simulink library "WiFi_lib"  (Simulink 5.0)
values from neighbouring files (symbols this model uses):
  cck_codes_11 = [1 1 1 -1 1 1 -1 1 -1 1 -1 -1 ... (512 elements, 8x64)]    [cck_codes.mat]
  cck_codes_55 = [6.12303176911e-17 1 6.12303176911e-17 -1 6.12303176911e-17 1 -6.12303176911e-17 1 -1.83690953073e-16 1 -1.83690953073e-16 -1 ... (32 elements, 8x4)]    [cck_codes.mat]
  Center_frequency = (Channel_number-6) *5    [WiFi_init.m]
  Channel_size_change = 0    [WiFi_init.m]
  Correction_delay = evalin('base', 'Correction_delay')    [WiFi_init.m]
  Spreading_rate = evalin('base','Spreading_rate')    [WiFi_init.m]
undefined symbols (not defined in the file or in its folder): Buffering_delay, Chip_rate, PLCP_header_size, PLCP_preamble_size, PLCP_size, PLCP_size_symbols, PPDU_frame_period, PPDU_size_symbols, PSDU_size, PSDU_size_symbols
libraries: simulink x46, commdigbbndpm2 x17, dspsigattribs x14, simulink3 x14, WiFi_lib x14, dspmathops x8, dspmtrx3 x6, dspindex x4, dspsrcs3 x3, dspstat3 x2, commdigbbndfm2 x2, commchan2 x1
settings Model: Creator=stuartm  LastModifiedBy=stuartm

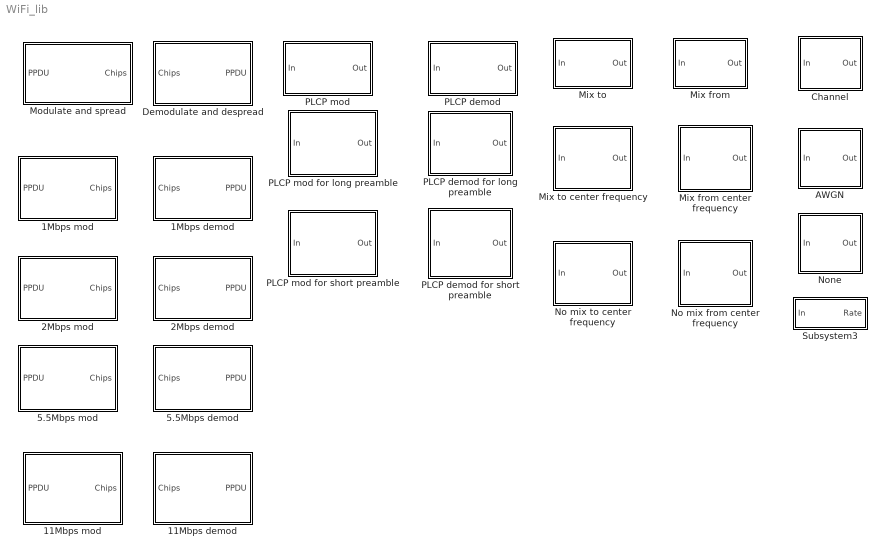
== system WiFi_lib ==
  11Mbps demod : Subsystem  mask{Short_preamble=off}
      mask prompts: Short_preamble "Short Preamble"
      mask init:
      | if Short_preamble
      |  set_param([gcb '/PLCP demod'],'BlockChoice','PLCP demod for short preamble')
      | else
      |   set_param([gcb '/PLCP demod'],'BlockChoice','PLCP demod for long preamble')
      | end
  11Mbps mod : Subsystem  mask{Short_preamble=off}
      mask prompts: Short_preamble "Short Preamble"
      mask init:
      | if Short_preamble
      |  set_param([gcb '/PLCP mod'],'BlockChoice','PLCP mod for short preamble')
      | else
      |   set_param([gcb '/PLCP mod'],'BlockChoice','PLCP mod for long preamble')
      | end
  1Mbps demod : Subsystem
  1Mbps mod : Subsystem
  2Mbps demod : Subsystem  mask{Short_preamble=off}
      mask prompts: Short_preamble "Short Preamble"
      mask init:
      | if Short_preamble
      |  set_param([gcb '/PLCP demod'],'BlockChoice','PLCP demod for short preamble')
      | else
      |   set_param([gcb '/PLCP demod'],'BlockChoice','PLCP demod for long preamble')
      | end
  2Mbps mod : Subsystem  mask{Short_preamble=off}
      mask prompts: Short_preamble "Short Preamble"
      mask init:
      | if Short_preamble
      |  set_param([gcb '/PLCP mod'],'BlockChoice','PLCP mod for short preamble')
      | else
      |   set_param([gcb '/PLCP mod'],'BlockChoice','PLCP mod for long preamble')
      | end
  5.5Mbps demod : Subsystem  mask{Short_preamble=off}
      mask prompts: Short_preamble "Short Preamble"
      mask init:
      | if Short_preamble
      |  set_param([gcb '/PLCP demod'],'BlockChoice','PLCP demod for short preamble')
      | else
      |   set_param([gcb '/PLCP demod'],'BlockChoice','PLCP demod for long preamble')
      | end
  5.5Mbps mod : Subsystem  mask{Short_preamble=off}
      mask prompts: Short_preamble "Short Preamble"
      mask init:
      | if Short_preamble
      |  set_param([gcb '/PLCP mod'],'BlockChoice','PLCP mod for short preamble')
      | else
      |   set_param([gcb '/PLCP mod'],'BlockChoice','PLCP mod for long preamble')
      | end
  AWGN : Subsystem
      mask Display: disp('Channel')
  Channel : Subsystem  BlockChoice=AWGN
      settings: TemplateBlock=self  MemberBlocks=AWGN,None
  Demodulate and despread : Subsystem  BlockChoice=11Mbps demod
      settings: TemplateBlock=self  MemberBlocks=11Mbps demod,1Mbps demod,2Mbps demod,5.5Mbps demod
  Mix from : Subsystem  BlockChoice=Mix from center frequency
      settings: TemplateBlock=self  MemberBlocks=Mix from center frequency,No mix from center frequency
  Mix from center frequency : Subsystem
  Mix to : Subsystem  BlockChoice=Mix to center frequency
      settings: TemplateBlock=self  MemberBlocks=Mix to center frequency,No mix to center frequency
  Mix to center frequency : Subsystem
  Modulate and spread : Subsystem  BlockChoice=11Mbps mod
      settings: TemplateBlock=self  MemberBlocks=11Mbps mod,1Mbps mod,2Mbps mod,5.5Mbps mod
  No mix from center frequency : Subsystem
  No mix to center frequency : Subsystem
  None : Subsystem
      mask Display: disp('Channel')
  PLCP demod : Subsystem  BlockChoice=PLCP demod for long preamble
      settings: TemplateBlock=self  MemberBlocks=PLCP demod for long preamble,PLCP demod for short preamble
  PLCP demod for long preamble : Subsystem
  PLCP demod for short preamble : Subsystem
  PLCP mod : Subsystem  BlockChoice=PLCP mod for long preamble
      settings: TemplateBlock=self  MemberBlocks=PLCP mod for long preamble,PLCP mod for short preamble
  PLCP mod for long preamble : Subsystem
  PLCP mod for short preamble : Subsystem
  Subsystem3 : Subsystem  mask(Display sample rate for framebased signals){Units=MHz}
      mask init:
      | switch Units
      | case 1
      |      Units_string='Hz';
      | case 2
      |      Units_string='KHz';
      | case 3
      |      Units_string='MHz';
      | end
      mask StyleString: popup(Hz|KHz|MHz)
      mask Display: disp(['Rate (' Units_string ')'])

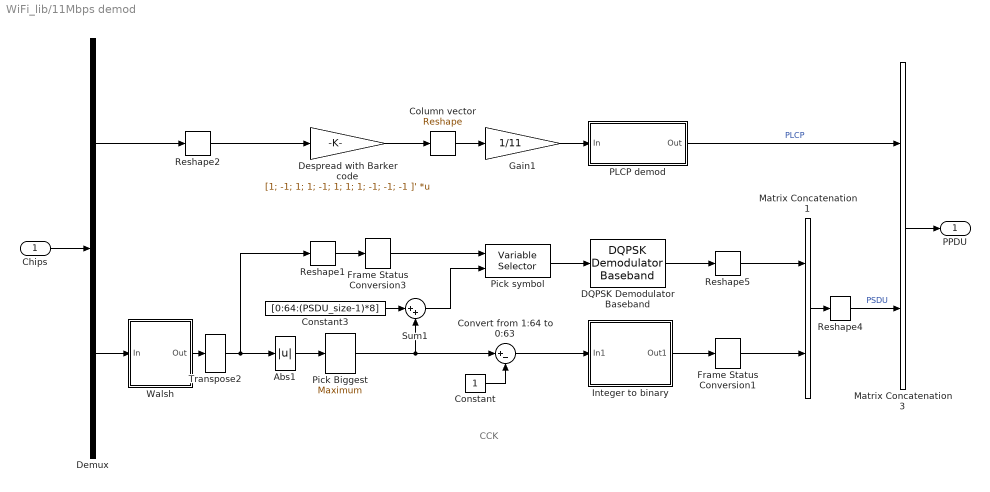
== system WiFi_lib/11Mbps demod ==
  note: CCK
  Chips : Inport
  Abs1 : Abs  SaturateOnIntegerOverflow=on
  Column vector : simulink/Math Operations/Reshape  OutputDimensionality=Column vector  OutputDimensions=[11,10]
  Constant : Constant
  Constant3 : Constant  Value=[0:64:(PSDU_size-1)*8]
  Convert from 1:64 to 0:63 : Sum  Inputs=|+-  SaturateOnIntegerOverflow=on  InputSameDT=on
  DQPSK Demodulator Baseband : commdigbbndpm2/DQPSK Demodulator Baseband  OutType=Bit  Dec=Binary  Ph=0  numSamp=1
  Demux : Demux  Outputs=[PLCP_size_symbols*Spreading_rate PSDU_size]
  Despread with Barker code : Gain  Gain=[1; -1; 1; 1; -1; 1; 1; 1; -1; -1; -1 ]'  Multiplication=Matrix(K*u)  SaturateOnIntegerOverflow=on
  Frame Status Conversion1 : dspsigattribs/Frame Status Conversion  growRefPort=off  outframe=Frame-based
  Frame Status Conversion3 : dspsigattribs/Frame Status Conversion  growRefPort=off  outframe=Frame-based
  Gain1 : Gain  Gain=1/11  SaturateOnIntegerOverflow=on
  Integer to binary : Subsystem
  Matrix Concatenation1 : simulink/Math Operations/Matrix Concatenation  numInports=2  catMethod=Vertical
  Matrix Concatenation3 : simulink/Math Operations/Matrix Concatenation  numInports=2  catMethod=Vertical
  PLCP demod : Subsystem  BlockChoice=PLCP demod for long preamble
      settings: AttributesFormatString=%<BlockChoice>  TemplateBlock=WiFi_lib/PLCP demod  MemberBlocks=PLCP demod for long preamble,PLCP demod for short preamble
  Pick Biggest : dspstat3/Maximum  fcn=Index  reset=None
  Pick symbol : dspindex/Variable Selector  rowsOrCols=Rows  IdxMode=Variable  Elements=[1 3]  ZerOneIdxMode=One-based  errmode=Clip Index
  Reshape1 : simulink/Math Operations/Reshape  OutputDimensionality=1-D array  OutputDimensions=[Spreading_rate,PLCP_size_symbols]
  Reshape2 : simulink/Math Operations/Reshape  OutputDimensionality=Customize  OutputDimensions=[Spreading_rate,PLCP_size_symbols]
  Reshape4 : simulink/Math Operations/Reshape  OutputDimensionality=Column vector  OutputDimensions=[Spreading_rate,PLCP_size_symbols]
  Reshape5 : simulink/Math Operations/Reshape  OutputDimensionality=Customize  OutputDimensions=[2,PSDU_size/8]
  Sum1 : Sum  Inputs=|++  SaturateOnIntegerOverflow=on  InputSameDT=on
  Transpose2 : dspmtrx3/Transpose  Hermitian=off
  Walsh : Subsystem
  PPDU : Outport
  wires:
  Gain1/1 -> PLCP demod/1(In)
  Despread with Barker code/1 -> Column vector/1
  Column vector/1 -> Gain1/1
  Demux/1 -> Reshape2/1
  Demux/2 -> Walsh/1(In)
  Chips/1 -> Demux/1
  PLCP demod/1(Out) -> Matrix Concatenation3/1  "PLCP"
  Reshape4/1 -> Matrix Concatenation3/2  "PSDU"
  Matrix Concatenation3/1 -> PPDU/1
  Walsh/1(Out) -> Transpose2/1
  Transpose2/1 -> Abs1/1, Reshape1/1
  Abs1/1 -> Pick Biggest/1
  Pick Biggest/1 -> Convert from 1:64 to 0:63/1, Sum1/2
  Constant/1 -> Convert from 1:64 to 0:63/2
  Convert from 1:64 to 0:63/1 -> Integer to binary/1(In1)
  Integer to binary/1(Out1) -> Frame Status Conversion1/1
  Pick symbol/1 -> DQPSK Demodulator Baseband/1
  Reshape5/1 -> Matrix Concatenation1/1
  Reshape1/1 -> Frame Status Conversion3/1
  Sum1/1 -> Pick symbol/2
  Constant3/1 -> Sum1/1
  Frame Status Conversion1/1 -> Matrix Concatenation1/2
  Frame Status Conversion3/1 -> Pick symbol/1
  Matrix Concatenation1/1 -> Reshape4/1
  DQPSK Demodulator Baseband/1 -> Reshape5/1
  Reshape2/1 -> Despread with Barker code/1

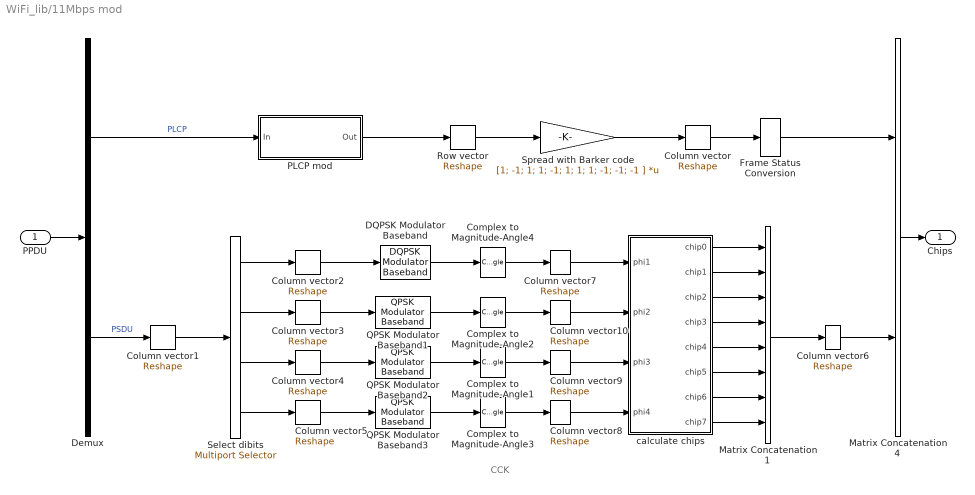
== system WiFi_lib/11Mbps mod ==
  note: CCK
  PPDU : Inport
  Column vector : simulink/Math Operations/Reshape  OutputDimensionality=Column vector  OutputDimensions=[1,1]
  Column vector1 : simulink/Math Operations/Reshape  OutputDimensionality=Customize  OutputDimensions=[8,PSDU_size/8]
  Column vector{7..10} (4 alike) : simulink/Math Operations/Reshape  OutputDimensionality=Row vector  OutputDimensions=[8,PSDU_size/8]
  Column vector{2..6} (5 alike) : simulink/Math Operations/Reshape  OutputDimensionality=Column vector  OutputDimensions=[8,PSDU_size/8]
  Complex to Magnitude-Angle{1..4} (4 alike) : ComplexToMagnitudeAngle  Output=Angle
  DQPSK Modulator Baseband : commdigbbndpm2/DQPSK Modulator Baseband  InType=Bit  Enc=Binary  Ph=0  numSamp=1
  Demux : Demux  Outputs=[PLCP_size PSDU_size]
  Frame Status Conversion : dspsigattribs/Frame Status Conversion  growRefPort=off  outframe=Frame-based
  Matrix Concatenation1 : simulink/Math Operations/Matrix Concatenation  numInports=8  catMethod=Vertical
  Matrix Concatenation4 : simulink/Math Operations/Matrix Concatenation  numInports=2  catMethod=Vertical
  PLCP mod : Subsystem  BlockChoice=PLCP mod for long preamble
      settings: AttributesFormatString=%<BlockChoice>  TemplateBlock=WiFi_lib/PLCP mod  MemberBlocks=PLCP mod for long preamble,PLCP mod for short preamble
  QPSK Modulator Baseband1 : commdigbbndpm2/QPSK Modulator Baseband  InType=Bit  Enc=Binary  Ph=0  numSamp=1
  QPSK Modulator Baseband2 : commdigbbndpm2/QPSK Modulator Baseband  InType=Bit  Enc=Binary  Ph=0  numSamp=1
  QPSK Modulator Baseband3 : commdigbbndpm2/QPSK Modulator Baseband  InType=Bit  Enc=Binary  Ph=0  numSamp=1
  Row vector : simulink/Math Operations/Reshape  OutputDimensionality=Row vector  OutputDimensions=[1,1]
  Select dibits : dspindex/Multiport Selector  rowsOrCols=Rows  idxCellArray={ [1 2], [3 4], [5 6], [ 7 8] }  idxErrMode=Generate Error
  Spread with Barker code : Gain  Gain=[1; -1; 1; 1; -1; 1; 1; 1; -1; -1; -1 ]  Multiplication=Matrix(K*u)  SaturateOnIntegerOverflow=on
  calculate chips : Subsystem
  Chips : Outport
  wires:
  Column vector6/1 -> Matrix Concatenation4/2
  PLCP mod/1(Out) -> Row vector/1
  Spread with Barker code/1 -> Column vector/1
  Column vector/1 -> Frame Status Conversion/1
  Frame Status Conversion/1 -> Matrix Concatenation4/1
  Matrix Concatenation4/1 -> Chips/1
  PPDU/1 -> Demux/1
  Demux/1 -> PLCP mod/1(In)  "PLCP"
  Demux/2 -> Column vector1/1  "PSDU"
  Column vector1/1 -> Select dibits/1
  Select dibits/1 -> Column vector2/1
  Select dibits/2 -> Column vector3/1
  Select dibits/3 -> Column vector4/1
  Select dibits/4 -> Column vector5/1
  Column vector2/1 -> DQPSK Modulator Baseband/1
  Column vector3/1 -> QPSK Modulator Baseband1/1
  Column vector4/1 -> QPSK Modulator Baseband2/1
  Column vector5/1 -> QPSK Modulator Baseband3/1
  DQPSK Modulator Baseband/1 -> Complex to Magnitude-Angle4/1
  QPSK Modulator Baseband1/1 -> Complex to Magnitude-Angle2/1
  QPSK Modulator Baseband2/1 -> Complex to Magnitude-Angle1/1
  QPSK Modulator Baseband3/1 -> Complex to Magnitude-Angle3/1
  Complex to Magnitude-Angle4/1 -> Column vector7/1
  Complex to Magnitude-Angle2/1 -> Column vector10/1
  Complex to Magnitude-Angle1/1 -> Column vector9/1
  Complex to Magnitude-Angle3/1 -> Column vector8/1
  calculate chips/2(chip1) -> Matrix Concatenation1/2
  calculate chips/3(chip2) -> Matrix Concatenation1/3
  calculate chips/4(chip3) -> Matrix Concatenation1/4
  calculate chips/5(chip4) -> Matrix Concatenation1/5
  calculate chips/6(chip5) -> Matrix Concatenation1/6
  calculate chips/7(chip6) -> Matrix Concatenation1/7
  calculate chips/8(chip7) -> Matrix Concatenation1/8
  Matrix Concatenation1/1 -> Column vector6/1
  Column vector8/1 -> calculate chips/4(phi4)
  Column vector9/1 -> calculate chips/3(phi3)
  Column vector10/1 -> calculate chips/2(phi2)
  Column vector7/1 -> calculate chips/1(phi1)
  calculate chips/1(chip0) -> Matrix Concatenation1/1
  Row vector/1 -> Spread with Barker code/1

== system WiFi_lib/1Mbps demod ==
  Chips : Inport
  Column vector : simulink/Math Operations/Reshape  OutputDimensionality=Column vector  OutputDimensions=[11,10]
  DBPSK Demodulator Baseband : commdigbbndpm2/DBPSK Demodulator Baseband  Ph=0  numSamp=1
  Despread with Barker code : Gain  Gain=[1; -1; 1; 1; -1; 1; 1; 1; -1; -1; -1 ]'  Multiplication=Matrix(K*u)  SaturateOnIntegerOverflow=on
  Gain1 : Gain  Gain=1/11  SaturateOnIntegerOverflow=on
  Reshape2 : simulink/Math Operations/Reshape  OutputDimensionality=Customize  OutputDimensions=[Spreading_rate,PPDU_size_symbols]
  PPDU : Outport
  wires:
  DBPSK Demodulator Baseband/1 -> PPDU/1
  Chips/1 -> Reshape2/1
  Column vector/1 -> Gain1/1
  Despread with Barker code/1 -> Column vector/1
  Gain1/1 -> DBPSK Demodulator Baseband/1
  Reshape2/1 -> Despread with Barker code/1

== system WiFi_lib/1Mbps mod ==
  PPDU : Inport
  Column vector : simulink/Math Operations/Reshape  OutputDimensionality=Column vector  OutputDimensions=[1,1]
  DBPSK Modulator Baseband1 : commdigbbndpm2/DBPSK Modulator Baseband  Ph=0  numSamp=1
  Frame Status Conversion : dspsigattribs/Frame Status Conversion  growRefPort=off  outframe=Frame-based
  Row vector : simulink/Math Operations/Reshape  OutputDimensionality=Row vector  OutputDimensions=[1,1]
  Spread with Barker code : Gain  Gain=[1; -1; 1; 1; -1; 1; 1; 1; -1; -1; -1 ]  Multiplication=Matrix(K*u)  SaturateOnIntegerOverflow=on
  Chips : Outport
  wires:
  DBPSK Modulator Baseband1/1 -> Row vector/1
  Spread with Barker code/1 -> Column vector/1
  Column vector/1 -> Frame Status Conversion/1  "PPDU"
  PPDU/1 -> DBPSK Modulator Baseband1/1
  Frame Status Conversion/1 -> Chips/1  "PPDU"
  Row vector/1 -> Spread with Barker code/1

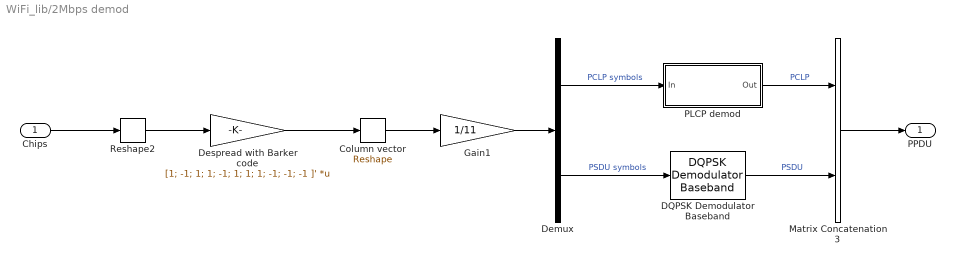
== system WiFi_lib/2Mbps demod ==
  Chips : Inport
  Column vector : simulink/Math Operations/Reshape  OutputDimensionality=Column vector  OutputDimensions=[11,10]
  DQPSK Demodulator Baseband : commdigbbndpm2/DQPSK Demodulator Baseband  OutType=Bit  Dec=Gray  Ph=0  numSamp=1
  Demux : Demux  Outputs=[PLCP_size_symbols PSDU_size_symbols]
  Despread with Barker code : Gain  Gain=[1; -1; 1; 1; -1; 1; 1; 1; -1; -1; -1 ]'  Multiplication=Matrix(K*u)  SaturateOnIntegerOverflow=on
  Gain1 : Gain  Gain=1/11  SaturateOnIntegerOverflow=on
  Matrix Concatenation3 : simulink/Math Operations/Matrix Concatenation  numInports=2  catMethod=Vertical
  PLCP demod : Subsystem  BlockChoice=PLCP demod for long preamble
      settings: AttributesFormatString=%<BlockChoice>  TemplateBlock=WiFi_lib/PLCP demod  MemberBlocks=PLCP demod for long preamble,PLCP demod for short preamble
  Reshape2 : simulink/Math Operations/Reshape  OutputDimensionality=Customize  OutputDimensions=[Spreading_rate,PPDU_size_symbols]
  PPDU : Outport
  wires:
  PLCP demod/1(Out) -> Matrix Concatenation3/1  "PCLP"
  Demux/1 -> PLCP demod/1(In)  "PCLP symbols"
  Demux/2 -> DQPSK Demodulator Baseband/1  "PSDU symbols"
  Gain1/1 -> Demux/1
  Despread with Barker code/1 -> Column vector/1
  Column vector/1 -> Gain1/1
  Chips/1 -> Reshape2/1
  Matrix Concatenation3/1 -> PPDU/1
  DQPSK Demodulator Baseband/1 -> Matrix Concatenation3/2  "PSDU"
  Reshape2/1 -> Despread with Barker code/1

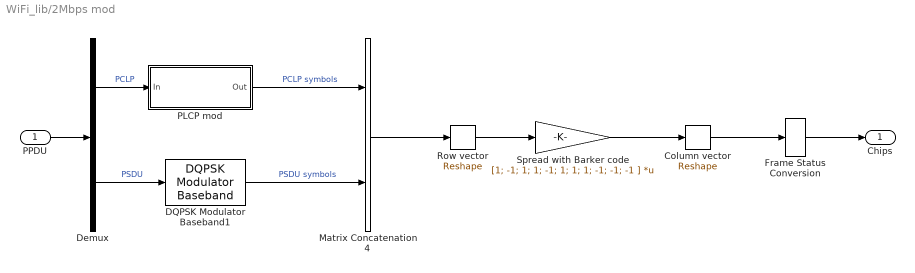
== system WiFi_lib/2Mbps mod ==
  PPDU : Inport
  Column vector : simulink/Math Operations/Reshape  OutputDimensionality=Column vector  OutputDimensions=[1,1]
  DQPSK Modulator Baseband1 : commdigbbndpm2/DQPSK Modulator Baseband  InType=Bit  Enc=Gray  Ph=0  numSamp=1
  Demux : Demux  Outputs=[PLCP_size PSDU_size]
  Frame Status Conversion : dspsigattribs/Frame Status Conversion  growRefPort=off  outframe=Frame-based
  Matrix Concatenation4 : simulink/Math Operations/Matrix Concatenation  numInports=2  catMethod=Vertical
  PLCP mod : Subsystem  BlockChoice=PLCP mod for long preamble
      settings: AttributesFormatString=%<BlockChoice>  TemplateBlock=WiFi_lib/PLCP mod  MemberBlocks=PLCP mod for long preamble,PLCP mod for short preamble
  Row vector : simulink/Math Operations/Reshape  OutputDimensionality=Row vector  OutputDimensions=[1,1]
  Spread with Barker code : Gain  Gain=[1; -1; 1; 1; -1; 1; 1; 1; -1; -1; -1 ]  Multiplication=Matrix(K*u)  SaturateOnIntegerOverflow=on
  Chips : Outport
  wires:
  Spread with Barker code/1 -> Column vector/1
  Column vector/1 -> Frame Status Conversion/1
  Frame Status Conversion/1 -> Chips/1
  PLCP mod/1(Out) -> Matrix Concatenation4/1  "PCLP symbols"
  Matrix Concatenation4/1 -> Row vector/1
  DQPSK Modulator Baseband1/1 -> Matrix Concatenation4/2  "PSDU symbols"
  Demux/1 -> PLCP mod/1(In)  "PCLP"
  PPDU/1 -> Demux/1
  Demux/2 -> DQPSK Modulator Baseband1/1  "PSDU"
  Row vector/1 -> Spread with Barker code/1

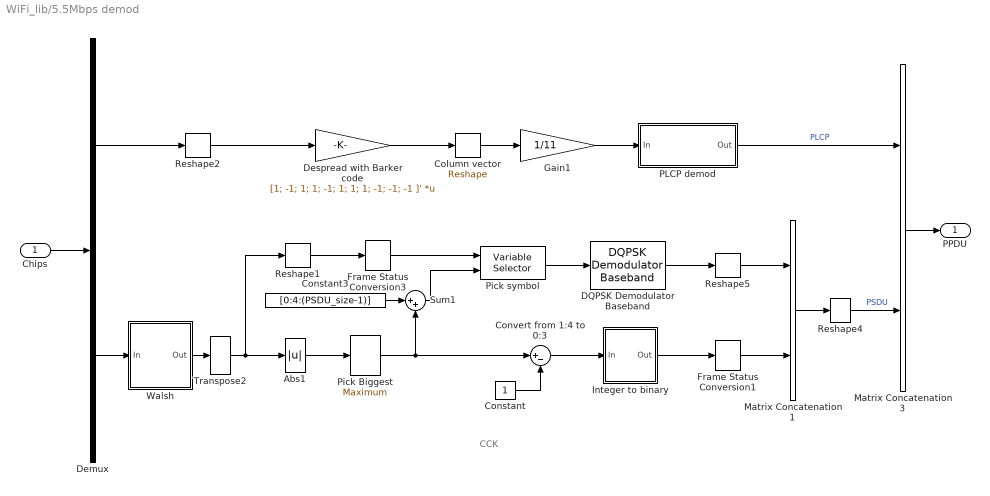
== system WiFi_lib/5.5Mbps demod ==
  note: CCK
  Chips : Inport
  Abs1 : Abs  SaturateOnIntegerOverflow=on
  Column vector : simulink/Math Operations/Reshape  OutputDimensionality=Column vector  OutputDimensions=[11,10]
  Constant : Constant
  Constant3 : Constant  Value=[0:4:(PSDU_size-1)]
  Convert from 1:4 to 0:3 : Sum  Inputs=|+-  SaturateOnIntegerOverflow=on  InputSameDT=on
  DQPSK Demodulator Baseband : commdigbbndpm2/DQPSK Demodulator Baseband  OutType=Bit  Dec=Binary  Ph=0  numSamp=1
  Demux : Demux  Outputs=[PLCP_size_symbols*Spreading_rate PSDU_size*2]
  Despread with Barker code : Gain  Gain=[1; -1; 1; 1; -1; 1; 1; 1; -1; -1; -1 ]'  Multiplication=Matrix(K*u)  SaturateOnIntegerOverflow=on
  Frame Status Conversion1 : dspsigattribs/Frame Status Conversion  growRefPort=off  outframe=Frame-based
  Frame Status Conversion3 : dspsigattribs/Frame Status Conversion  growRefPort=off  outframe=Frame-based
  Gain1 : Gain  Gain=1/11  SaturateOnIntegerOverflow=on
  Integer to binary : Subsystem
  Matrix Concatenation1 : simulink/Math Operations/Matrix Concatenation  numInports=2  catMethod=Vertical
  Matrix Concatenation3 : simulink/Math Operations/Matrix Concatenation  numInports=2  catMethod=Vertical
  PLCP demod : Subsystem  BlockChoice=PLCP demod for long preamble
      settings: AttributesFormatString=%<BlockChoice>  TemplateBlock=WiFi_lib/PLCP demod  MemberBlocks=PLCP demod for long preamble,PLCP demod for short preamble
  Pick Biggest : dspstat3/Maximum  fcn=Index  reset=None
  Pick symbol : dspindex/Variable Selector  rowsOrCols=Rows  IdxMode=Variable  Elements=[1 3]  ZerOneIdxMode=One-based  errmode=Clip Index
  Reshape1 : simulink/Math Operations/Reshape  OutputDimensionality=1-D array  OutputDimensions=[Spreading_rate,PLCP_size_symbols]
  Reshape2 : simulink/Math Operations/Reshape  OutputDimensionality=Customize  OutputDimensions=[Spreading_rate,PLCP_size_symbols]
  Reshape4 : simulink/Math Operations/Reshape  OutputDimensionality=Column vector  OutputDimensions=[Spreading_rate,PLCP_size_symbols]
  Reshape5 : simulink/Math Operations/Reshape  OutputDimensionality=Customize  OutputDimensions=[2,PSDU_size/4]
  Sum1 : Sum  Inputs=|++  SaturateOnIntegerOverflow=on  InputSameDT=on
  Transpose2 : dspmtrx3/Transpose  Hermitian=off
  Walsh : Subsystem
  PPDU : Outport
  wires:
  DQPSK Demodulator Baseband/1 -> Reshape5/1
  Matrix Concatenation1/1 -> Reshape4/1
  Frame Status Conversion3/1 -> Pick symbol/1
  Frame Status Conversion1/1 -> Matrix Concatenation1/2
  Constant3/1 -> Sum1/1
  Sum1/1 -> Pick symbol/2
  Reshape1/1 -> Frame Status Conversion3/1
  Reshape5/1 -> Matrix Concatenation1/1
  Pick symbol/1 -> DQPSK Demodulator Baseband/1
  Integer to binary/1(Out) -> Frame Status Conversion1/1
  Convert from 1:4 to 0:3/1 -> Integer to binary/1(In)
  Constant/1 -> Convert from 1:4 to 0:3/2
  Pick Biggest/1 -> Sum1/2, Convert from 1:4 to 0:3/1
  Abs1/1 -> Pick Biggest/1
  Transpose2/1 -> Abs1/1, Reshape1/1
  Walsh/1(Out) -> Transpose2/1
  Matrix Concatenation3/1 -> PPDU/1
  Reshape4/1 -> Matrix Concatenation3/2  "PSDU"
  PLCP demod/1(Out) -> Matrix Concatenation3/1  "PLCP"
  Chips/1 -> Demux/1
  Demux/2 -> Walsh/1(In)
  Demux/1 -> Reshape2/1
  Column vector/1 -> Gain1/1
  Despread with Barker code/1 -> Column vector/1
  Gain1/1 -> PLCP demod/1(In)
  Reshape2/1 -> Despread with Barker code/1

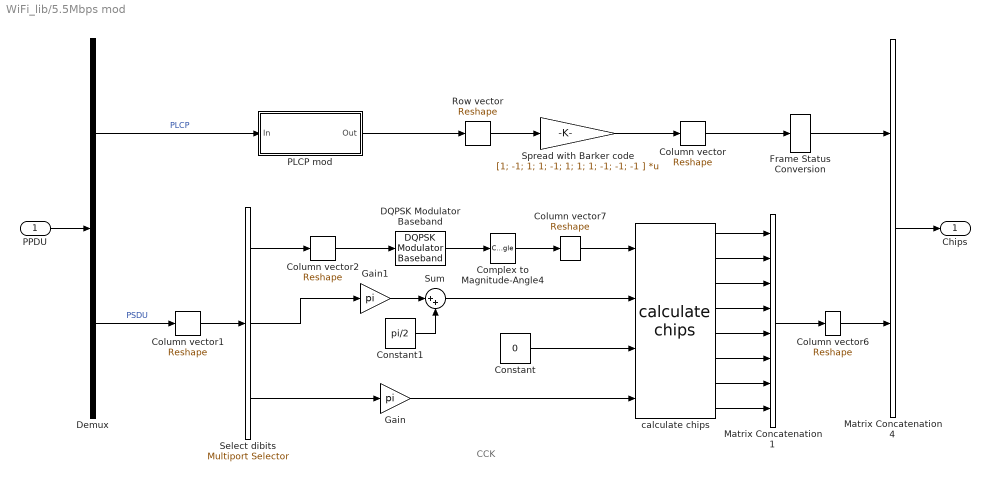
== system WiFi_lib/5.5Mbps mod ==
  note: CCK
  PPDU : Inport
  Column vector : simulink/Math Operations/Reshape  OutputDimensionality=Column vector  OutputDimensions=[1,1]
  Column vector1 : simulink/Math Operations/Reshape  OutputDimensionality=Customize  OutputDimensions=[4,PSDU_size/4]
  Column vector2 : simulink/Math Operations/Reshape  OutputDimensionality=Column vector  OutputDimensions=[8,PSDU_size/8]
  Column vector6 : simulink/Math Operations/Reshape  OutputDimensionality=Column vector  OutputDimensions=[8,PSDU_size/8]
  Column vector7 : simulink/Math Operations/Reshape  OutputDimensionality=Row vector  OutputDimensions=[8,PSDU_size/8]
  Complex to Magnitude-Angle4 : ComplexToMagnitudeAngle  Output=Angle
  Constant : Constant  Value=0
  Constant1 : Constant  Value=pi/2
  DQPSK Modulator Baseband : commdigbbndpm2/DQPSK Modulator Baseband  InType=Bit  Enc=Binary  Ph=0  numSamp=1
  Demux : Demux  Outputs=[PLCP_size PSDU_size]
  Frame Status Conversion : dspsigattribs/Frame Status Conversion  growRefPort=off  outframe=Frame-based
  Gain : Gain  Gain=pi  SaturateOnIntegerOverflow=on
  Gain1 : Gain  Gain=pi  SaturateOnIntegerOverflow=on
  Matrix Concatenation1 : simulink/Math Operations/Matrix Concatenation  numInports=8  catMethod=Vertical
  Matrix Concatenation4 : simulink/Math Operations/Matrix Concatenation  numInports=2  catMethod=Vertical
  PLCP mod : Subsystem  BlockChoice=PLCP mod for long preamble
      settings: AttributesFormatString=%<BlockChoice>  TemplateBlock=WiFi_lib/PLCP mod  MemberBlocks=PLCP mod for long preamble,PLCP mod for short preamble
  Row vector : simulink/Math Operations/Reshape  OutputDimensionality=Row vector  OutputDimensions=[1,1]
  Select dibits : dspindex/Multiport Selector  rowsOrCols=Rows  idxCellArray={ [1 2], 3,4}  idxErrMode=Generate Error
  Spread with Barker code : Gain  Gain=[1; -1; 1; 1; -1; 1; 1; 1; -1; -1; -1 ]  Multiplication=Matrix(K*u)  SaturateOnIntegerOverflow=on
  Sum : Sum  Inputs=|++  SaturateOnIntegerOverflow=on  InputSameDT=on
  calculate chips : WiFi_lib/11Mbps mod/calculate chips  SimViewingDevice=off  DataTypeOverride=UseLocalSettings  MinMaxOverflowLogging=UseLocalSettings
      settings: Permissions=ReadWrite  RTWFcnNameOpts=Auto  RTWFileNameOpts=Auto
  Chips : Outport
  wires:
  Column vector6/1 -> Matrix Concatenation4/2
  PLCP mod/1(Out) -> Row vector/1
  Demux/1 -> PLCP mod/1(In)  "PLCP"
  Spread with Barker code/1 -> Column vector/1
  Column vector/1 -> Frame Status Conversion/1
  Frame Status Conversion/1 -> Matrix Concatenation4/1
  Matrix Concatenation4/1 -> Chips/1
  Demux/2 -> Column vector1/1  "PSDU"
  PPDU/1 -> Demux/1
  Column vector1/1 -> Select dibits/1
  Select dibits/1 -> Column vector2/1
  Column vector2/1 -> DQPSK Modulator Baseband/1
  DQPSK Modulator Baseband/1 -> Complex to Magnitude-Angle4/1
  Complex to Magnitude-Angle4/1 -> Column vector7/1
  calculate chips/2 -> Matrix Concatenation1/2
  calculate chips/3 -> Matrix Concatenation1/3
  calculate chips/4 -> Matrix Concatenation1/4
  calculate chips/5 -> Matrix Concatenation1/5
  calculate chips/6 -> Matrix Concatenation1/6
  calculate chips/7 -> Matrix Concatenation1/7
  calculate chips/8 -> Matrix Concatenation1/8
  Matrix Concatenation1/1 -> Column vector6/1
  Column vector7/1 -> calculate chips/1
  calculate chips/1 -> Matrix Concatenation1/1
  Gain/1 -> calculate chips/4
  Constant/1 -> calculate chips/3
  Gain1/1 -> Sum/1
  Constant1/1 -> Sum/2
  Sum/1 -> calculate chips/2
  Select dibits/2 -> Gain1/1
  Select dibits/3 -> Gain/1
  Row vector/1 -> Spread with Barker code/1

== system WiFi_lib/AWGN ==
  In : Inport
  AWGN Channel : commchan2/AWGN Channel  seed=1237  noiseMode="Signal to noise ratio  (Es/No)"  EsNodB=EsNo  SNRdB=10  Ps=1  Tsym=1/Chip_rate  variance=1
  Out : Outport
  wires:
  AWGN Channel/1 -> Out/1
  In/1 -> AWGN Channel/1

== system WiFi_lib/Channel ==
  In : Inport
  AWGN : WiFi_lib/AWGN
  Out : Outport
  wires:
  In/1 -> AWGN/1
  AWGN/1 -> Out/1

== system WiFi_lib/Demodulate and despread ==
  Chips : Inport
  11Mbps demod : WiFi_lib/11Mbps demod  Short_preamble=off
  PPDU : Outport
  wires:
  Chips/1 -> 11Mbps demod/1
  11Mbps demod/1 -> PPDU/1

== system WiFi_lib/Mix from ==
  In : Inport
  Mix from center frequency : WiFi_lib/Mix from center frequency
      settings: RTWFcnNameOpts=Auto  RTWFileNameOpts=Auto
  Out : Outport
  wires:
  In/1 -> Mix from center frequency/1
  Mix from center frequency/1 -> Out/1

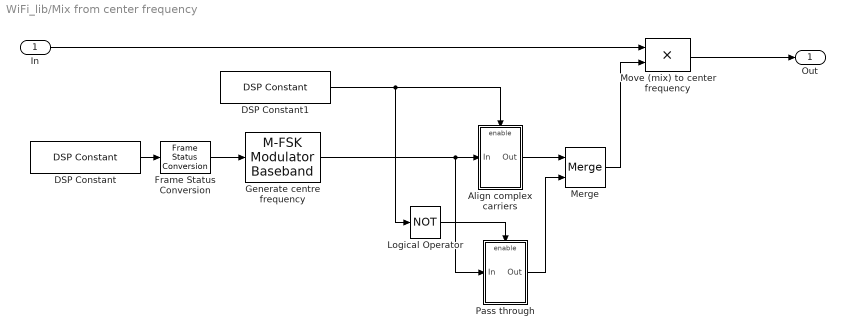
== system WiFi_lib/Mix from center frequency ==
  In : Inport
  Align complex carriers : Subsystem  TreatAsAtomicUnit=on
  DSP Constant : dspsrcs3/DSP Constant  Value=-Center_frequency+39  InterpretAs1D=off  SampleMode=Discrete  Ts=PPDU_frame_period/8  FramebasedOutput=off
  DSP Constant1 : dspsrcs3/DSP Constant  Value=Channel_size_change  InterpretAs1D=off  SampleMode=Discrete  Ts=PPDU_frame_period/8  FramebasedOutput=off
  Frame Status Conversion : dspsigattribs/Frame Status Conversion  growRefPort=off  outframe=Frame-based
  "Generate centre frequency " : commdigbbndfm2/M-FSK Modulator Baseband  M=79  InType=Integer  Enc=Binary  freqSep=1e6  phaseType=Continuous  numSamp=PPDU_size_chips
  Logical Operator : Logic  Operator=NOT
  Merge : Merge
  Move (mix) to center frequency : Product  SaturateOnIntegerOverflow=on  InputSameDT=on
  Pass through : Subsystem  TreatAsAtomicUnit=on
  Out : Outport
  wires:
  Frame Status Conversion/1 -> "Generate centre frequency "/1
  DSP Constant/1 -> Frame Status Conversion/1
  In/1 -> Move (mix) to center frequency/1
  Move (mix) to center frequency/1 -> Out/1
  "Generate centre frequency "/1 -> Align complex carriers/1(In), Pass through/1(In)
  DSP Constant1/1 -> Align complex carriers/Enable, Logical Operator/1
  Logical Operator/1 -> Pass through/Enable
  Align complex carriers/1(Out) -> Merge/1
  Pass through/1(Out) -> Merge/2
  Merge/1 -> Move (mix) to center frequency/2

== system WiFi_lib/Mix to ==
  In : Inport
  Mix to center frequency : WiFi_lib/Mix to center frequency
      settings: RTWFcnNameOpts=Auto  RTWFileNameOpts=Auto
  Out : Outport
  wires:
  In/1 -> Mix to center frequency/1
  Mix to center frequency/1 -> Out/1

== system WiFi_lib/Mix to center frequency ==
  In : Inport
  DSP Constant : dspsrcs3/DSP Constant  Value=Center_frequency+39  InterpretAs1D=off  SampleMode=Discrete  Ts=PPDU_frame_period/8  FramebasedOutput=off
  Frame Status Conversion : dspsigattribs/Frame Status Conversion  growRefPort=off  outframe=Frame-based
  "Generate centre frequency " : commdigbbndfm2/M-FSK Modulator Baseband  M=79  InType=Integer  Enc=Binary  freqSep=1e6  phaseType=Continuous  numSamp=PPDU_size_chips
  Move center frequency : Product  SaturateOnIntegerOverflow=on  InputSameDT=on
  Out : Outport
  wires:
  Move center frequency/1 -> Out/1
  In/1 -> Move center frequency/1
  DSP Constant/1 -> Frame Status Conversion/1
  "Generate centre frequency "/1 -> Move center frequency/2
  Frame Status Conversion/1 -> "Generate centre frequency "/1

== system WiFi_lib/Modulate and spread ==
  PPDU : Inport
  11Mbps mod : WiFi_lib/11Mbps mod  Short_preamble=off
  Chips : Outport
  wires:
  PPDU/1 -> 11Mbps mod/1
  11Mbps mod/1 -> Chips/1

== system WiFi_lib/No mix from center frequency ==
  In : Inport
  Out : Outport
  wires:
  In/1 -> Out/1

== system WiFi_lib/No mix to center frequency ==
  In : Inport
  Out : Outport
  wires:
  In/1 -> Out/1

== system WiFi_lib/None ==
  In : Inport
  Out : Outport
  wires:
  In/1 -> Out/1

== system WiFi_lib/PLCP demod ==
  In : Inport
  PLCP demod for long preamble : WiFi_lib/PLCP demod for long preamble
      settings: RTWFcnNameOpts=Auto  RTWFileNameOpts=Auto
  Out : Outport
  wires:
  In/1 -> PLCP demod for long preamble/1
  PLCP demod for long preamble/1 -> Out/1

== system WiFi_lib/PLCP demod for long preamble ==
  In : Inport
  DBPSK Demodulator Baseband : commdigbbndpm2/DBPSK Demodulator Baseband  Ph=0  numSamp=1
  Out : Outport
  wires:
  DBPSK Demodulator Baseband/1 -> Out/1
  In/1 -> DBPSK Demodulator Baseband/1  "PLCP"

== system WiFi_lib/PLCP demod for short preamble ==
  In : Inport
  DBPSK Demodulator Baseband : commdigbbndpm2/DBPSK Demodulator Baseband  Ph=0  numSamp=1
  DQPSK Demodulator Baseband : commdigbbndpm2/DQPSK Demodulator Baseband  OutType=Bit  Dec=Gray  Ph=0  numSamp=1
  Demux : Demux  Outputs=[PLCP_preamble_size PLCP_header_size/2]
  Matrix Concatenation4 : simulink3/Signals & Systems/Matrix Concatenation  numInports=2  catMethod=Vertical
  Out : Outport
  wires:
  In/1 -> Demux/1  "PLCP"
  Demux/2 -> DQPSK Demodulator Baseband/1
  Demux/1 -> DBPSK Demodulator Baseband/1
  DBPSK Demodulator Baseband/1 -> Matrix Concatenation4/1  "Preamble"
  DQPSK Demodulator Baseband/1 -> Matrix Concatenation4/2  "Header"
  Matrix Concatenation4/1 -> Out/1

== system WiFi_lib/PLCP mod ==
  In : Inport
  PLCP mod for long preamble : WiFi_lib/PLCP mod for long preamble
      settings: RTWFcnNameOpts=Auto  RTWFileNameOpts=Auto
  Out : Outport
  wires:
  In/1 -> PLCP mod for long preamble/1
  PLCP mod for long preamble/1 -> Out/1

== system WiFi_lib/PLCP mod for long preamble ==
  In : Inport
  DBPSK Modulator Baseband1 : commdigbbndpm2/DBPSK Modulator Baseband  Ph=0  numSamp=1
  Out : Outport
  wires:
  In/1 -> DBPSK Modulator Baseband1/1  "PLCP"
  DBPSK Modulator Baseband1/1 -> Out/1

== system WiFi_lib/PLCP mod for short preamble ==
  In : Inport
  DBPSK Modulator Baseband1 : commdigbbndpm2/DBPSK Modulator Baseband  Ph=0  numSamp=1
  DQPSK Modulator Baseband1 : commdigbbndpm2/DQPSK Modulator Baseband  InType=Bit  Enc=Gray  Ph=0  numSamp=1
  Demux : Demux  Outputs=[PLCP_preamble_size PLCP_header_size]
  Matrix Concatenation4 : simulink3/Signals & Systems/Matrix Concatenation  numInports=2  catMethod=Vertical
  Out : Outport
  wires:
  DBPSK Modulator Baseband1/1 -> Matrix Concatenation4/1
  Demux/1 -> DBPSK Modulator Baseband1/1  "Preamble"
  DQPSK Modulator Baseband1/1 -> Matrix Concatenation4/2
  Demux/2 -> DQPSK Modulator Baseband1/1  "Header"
  Matrix Concatenation4/1 -> Out/1
  In/1 -> Demux/1

== system WiFi_lib/Subsystem3 ==
  In : Inport
  Divide by rate units : Gain  Gain=1/10^((Units-1)*3)  SaturateOnIntegerOverflow=on
  Probe : Probe  ProbeWidth=off  ProbeComplexSignal=off  ProbeSignalDimensions=on
  Product : Product  Inputs=/*  SaturateOnIntegerOverflow=on  InputSameDT=on
  Selector : Selector  Elements=[1]  InputPortWidth=2
  Selector1 : Selector  Elements=[1]  InputPortWidth=2
  Rate : Outport
  wires:
  Divide by rate units/1 -> Rate/1
  Probe/1 -> Selector/1
  Probe/2 -> Selector1/1
  Selector/1 -> Product/1
  Selector1/1 -> Product/2
  In/1 -> Probe/1
  Product/1 -> Divide by rate units/1

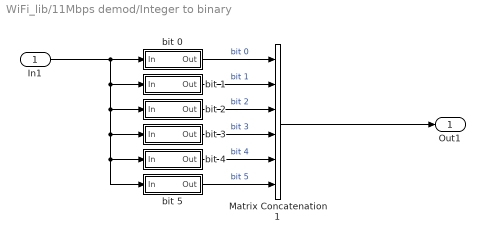
== system WiFi_lib/11Mbps demod/Integer to binary ==
  In1 : Inport
  Matrix Concatenation1 : simulink3/Signals & Systems/Matrix Concatenation  numInports=6  catMethod=Vertical
  bit 0 : Subsystem
  bit 1 : Subsystem
  bit 2 : Subsystem
  bit 3 : Subsystem
  bit 4 : Subsystem
  bit 5 : Subsystem
  Out1 : Outport
  wires:
  In1/1 -> bit 4/1(In), bit 5/1(In), bit 3/1(In), bit 2/1(In), bit 1/1(In), bit 0/1(In)
  bit 0/1(Out) -> Matrix Concatenation1/1  "bit 0"
  bit 1/1(Out) -> Matrix Concatenation1/2  "bit 1"
  bit 2/1(Out) -> Matrix Concatenation1/3  "bit 2"
  bit 3/1(Out) -> Matrix Concatenation1/4  "bit 3"
  bit 4/1(Out) -> Matrix Concatenation1/5  "bit 4"
  bit 5/1(Out) -> Matrix Concatenation1/6  "bit 5"
  Matrix Concatenation1/1 -> Out1/1

== system WiFi_lib/11Mbps demod/PLCP demod ==
  In : Inport
  PLCP demod for long preamble : WiFi_lib/PLCP demod for long preamble  SimViewingDevice=off  DataTypeOverride=UseLocalSettings  MinMaxOverflowLogging=UseLocalSettings
      settings: Permissions=ReadWrite  RTWFcnNameOpts=Auto  RTWFileNameOpts=Auto
  Out : Outport
  wires:
  In/1 -> PLCP demod for long preamble/1
  PLCP demod for long preamble/1 -> Out/1

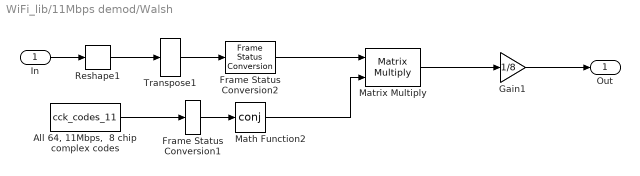
== system WiFi_lib/11Mbps demod/Walsh ==
  In : Inport
  "All 64, 11Mbps,  8 chip complex codes" : Constant  Value=cck_codes_11
  Frame Status Conversion1 : dspsigattribs/Frame Status Conversion  growRefPort=off  outframe=Frame-based
  Frame Status Conversion2 : dspsigattribs/Frame Status Conversion  growRefPort=off  outframe=Frame-based
  Gain1 : Gain  Gain=1/8  SaturateOnIntegerOverflow=on
  Math Function2 : Math  Operator=conj
  Matrix Multiply : dspmtrx3/Matrix Multiply  numInputPorts=2  OptimizationLevel=None
  Reshape1 : simulink3/Signals & Systems/Reshape  OutputDimensionality=Customize  OutputDimensions=[8,PSDU_size/8 ]
  Transpose1 : dspmtrx3/Transpose  Hermitian=off
  Out : Outport
  wires:
  "All 64, 11Mbps,  8 chip complex codes"/1 -> Frame Status Conversion1/1
  Reshape1/1 -> Transpose1/1
  Transpose1/1 -> Frame Status Conversion2/1
  Frame Status Conversion2/1 -> Matrix Multiply/1
  Frame Status Conversion1/1 -> Math Function2/1
  Math Function2/1 -> Matrix Multiply/2
  In/1 -> Reshape1/1
  Matrix Multiply/1 -> Gain1/1
  Gain1/1 -> Out/1

== system WiFi_lib/11Mbps mod/PLCP mod ==
  In : Inport
  PLCP mod for long preamble : WiFi_lib/PLCP mod for long preamble  SimViewingDevice=off  DataTypeOverride=UseLocalSettings  MinMaxOverflowLogging=UseLocalSettings
      settings: Permissions=ReadWrite  RTWFcnNameOpts=Auto  RTWFileNameOpts=Auto
  Out : Outport
  wires:
  In/1 -> PLCP mod for long preamble/1
  PLCP mod for long preamble/1 -> Out/1

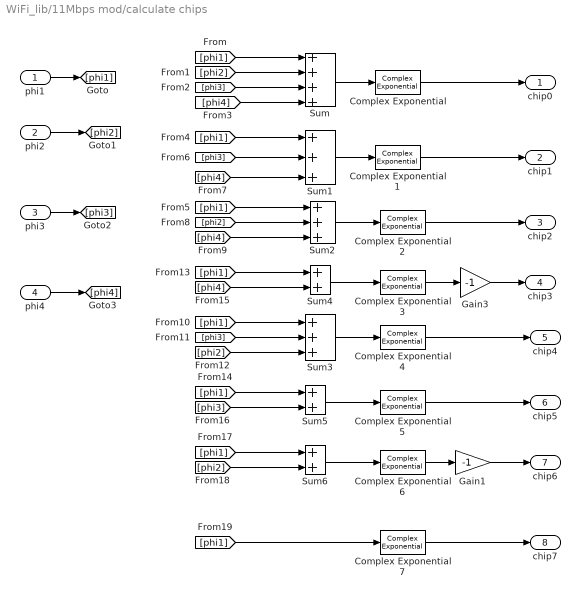
== system WiFi_lib/11Mbps mod/calculate chips ==
  phi1 : Inport
  phi2 : Inport  Port=2
  phi3 : Inport  Port=3
  phi4 : Inport  Port=4
  Complex Exponential{,1..7} (8 alike) : dspmathops/Complex Exponential
  Gain1 : Gain  Gain=-1  SaturateOnIntegerOverflow=on
  Gain3 : Gain  Gain=-1  SaturateOnIntegerOverflow=on
  Sum : Sum  Inputs=++++  SaturateOnIntegerOverflow=on  InputSameDT=on
  Sum1 : Sum  Inputs=+++  SaturateOnIntegerOverflow=on  InputSameDT=on
  Sum2 : Sum  Inputs=+++  SaturateOnIntegerOverflow=on  InputSameDT=on
  Sum3 : Sum  Inputs=+++  SaturateOnIntegerOverflow=on  InputSameDT=on
  Sum4 : Sum  SaturateOnIntegerOverflow=on  InputSameDT=on
  Sum5 : Sum  SaturateOnIntegerOverflow=on  InputSameDT=on
  Sum6 : Sum  SaturateOnIntegerOverflow=on  InputSameDT=on
  chip0 : Outport
  chip1 : Outport  Port=2
  chip2 : Outport  Port=3
  chip3 : Outport  Port=4
  chip4 : Outport  Port=5
  chip5 : Outport  Port=6
  chip6 : Outport  Port=7
  chip7 : Outport  Port=8
  wires:
  Sum/1 -> Complex Exponential/1
  Complex Exponential/1 -> chip0/1
  Complex Exponential1/1 -> chip1/1
  Complex Exponential2/1 -> chip2/1
  Complex Exponential3/1 -> Gain3/1
  Complex Exponential4/1 -> chip4/1
  Complex Exponential5/1 -> chip5/1
  Complex Exponential6/1 -> Gain1/1
  Complex Exponential7/1 -> chip7/1
  phi4/1 -> [phi4]
  phi3/1 -> [phi3]
  phi2/1 -> [phi2]
  phi1/1 -> [phi1]
  [phi1] -> Sum/1
  [phi2] -> Sum/2
  [phi3] -> Sum/3
  [phi4] -> Sum/4
  [phi1] -> Sum1/1
  [phi3] -> Sum1/2
  [phi4] -> Sum1/3
  Sum1/1 -> Complex Exponential1/1
  [phi1] -> Sum2/1
  [phi2] -> Sum2/2
  [phi4] -> Sum2/3
  Sum2/1 -> Complex Exponential2/1
  [phi1] -> Sum3/1
  [phi3] -> Sum3/2
  [phi2] -> Sum3/3
  Sum3/1 -> Complex Exponential4/1
  [phi1] -> Sum4/1
  [phi4] -> Sum4/2
  Sum4/1 -> Complex Exponential3/1
  [phi1] -> Sum5/1
  [phi3] -> Sum5/2
  Sum5/1 -> Complex Exponential5/1
  [phi1] -> Sum6/1
  [phi2] -> Sum6/2
  Sum6/1 -> Complex Exponential6/1
  [phi1] -> Complex Exponential7/1
  Gain3/1 -> chip3/1
  Gain1/1 -> chip6/1

== system WiFi_lib/2Mbps demod/PLCP demod ==
  In : Inport
  PLCP demod for long preamble : WiFi_lib/PLCP demod for long preamble  SimViewingDevice=off  DataTypeOverride=UseLocalSettings  MinMaxOverflowLogging=UseLocalSettings
      settings: Permissions=ReadWrite  RTWFcnNameOpts=Auto  RTWFileNameOpts=Auto
  Out : Outport
  wires:
  In/1 -> PLCP demod for long preamble/1
  PLCP demod for long preamble/1 -> Out/1

== system WiFi_lib/2Mbps mod/PLCP mod ==
  In : Inport
  PLCP mod for long preamble : WiFi_lib/PLCP mod for long preamble  SimViewingDevice=off  DataTypeOverride=UseLocalSettings  MinMaxOverflowLogging=UseLocalSettings
      settings: Permissions=ReadWrite  RTWFcnNameOpts=Auto  RTWFileNameOpts=Auto
  Out : Outport
  wires:
  In/1 -> PLCP mod for long preamble/1
  PLCP mod for long preamble/1 -> Out/1

== system WiFi_lib/5.5Mbps demod/Integer to binary ==
  In : Inport
  Matrix Concatenation1 : simulink3/Signals & Systems/Matrix Concatenation  numInports=2  catMethod=Vertical
  bit 0 : Subsystem
  bit 1 : Subsystem
  Out : Outport
  wires:
  Matrix Concatenation1/1 -> Out/1
  bit 1/1(Out) -> Matrix Concatenation1/2  "bit 1"
  bit 0/1(Out) -> Matrix Concatenation1/1  "bit 0"
  In/1 -> bit 0/1(In), bit 1/1(In)

== system WiFi_lib/5.5Mbps demod/PLCP demod ==
  In : Inport
  PLCP demod for long preamble : WiFi_lib/PLCP demod for long preamble  SimViewingDevice=off  DataTypeOverride=UseLocalSettings  MinMaxOverflowLogging=UseLocalSettings
      settings: Permissions=ReadWrite  RTWFcnNameOpts=Auto  RTWFileNameOpts=Auto
  Out : Outport
  wires:
  In/1 -> PLCP demod for long preamble/1
  PLCP demod for long preamble/1 -> Out/1

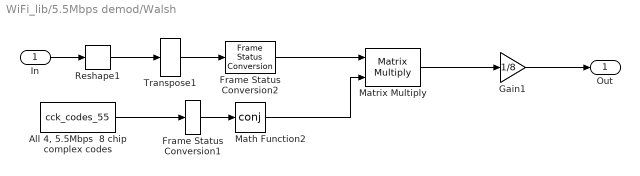
== system WiFi_lib/5.5Mbps demod/Walsh ==
  In : Inport
  "All 4, 5.5Mbps  8 chip complex codes" : Constant  Value=cck_codes_55
  Frame Status Conversion1 : dspsigattribs/Frame Status Conversion  growRefPort=off  outframe=Frame-based
  Frame Status Conversion2 : dspsigattribs/Frame Status Conversion  growRefPort=off  outframe=Frame-based
  Gain1 : Gain  Gain=1/8  SaturateOnIntegerOverflow=on
  Math Function2 : Math  Operator=conj
  Matrix Multiply : dspmtrx3/Matrix Multiply  numInputPorts=2  OptimizationLevel=None
  Reshape1 : simulink3/Signals & Systems/Reshape  OutputDimensionality=Customize  OutputDimensions=[8,PSDU_size/4 ]
  Transpose1 : dspmtrx3/Transpose  Hermitian=off
  Out : Outport
  wires:
  Gain1/1 -> Out/1
  Matrix Multiply/1 -> Gain1/1
  In/1 -> Reshape1/1
  Math Function2/1 -> Matrix Multiply/2
  Frame Status Conversion1/1 -> Math Function2/1
  Frame Status Conversion2/1 -> Matrix Multiply/1
  Transpose1/1 -> Frame Status Conversion2/1
  Reshape1/1 -> Transpose1/1
  "All 4, 5.5Mbps  8 chip complex codes"/1 -> Frame Status Conversion1/1

== system WiFi_lib/5.5Mbps mod/PLCP mod ==
  In : Inport
  PLCP mod for long preamble : WiFi_lib/PLCP mod for long preamble  SimViewingDevice=off  DataTypeOverride=UseLocalSettings  MinMaxOverflowLogging=UseLocalSettings
      settings: Permissions=ReadWrite  RTWFcnNameOpts=Auto  RTWFileNameOpts=Auto
  Out : Outport
  wires:
  In/1 -> PLCP mod for long preamble/1
  PLCP mod for long preamble/1 -> Out/1

== system WiFi_lib/Mix from center frequency/Align complex carriers ==
  In : Inport
  Enable : EnablePort
  Buffering correction : dspsigops/Integer Delay  delay=Channel_size_change*(Buffering_delay+Correction_delay)  ic=0
  Out : Outport
  wires:
  Buffering correction/1 -> Out/1
  In/1 -> Buffering correction/1

== system WiFi_lib/Mix from center frequency/Pass through ==
  In : Inport
  Enable : EnablePort
  Out : Outport
  wires:
  In/1 -> Out/1

== system WiFi_lib/11Mbps demod/Integer to binary/bit 0 ==
  In : Inport
  Bitwise Logical Operator : simulink3/Math/Bitwise Logical Operator  Operator=AND  Operand2=1
  Constant1 : Constant  Value=0
  Data Type Conversion : DataTypeConversion  DataType=uint8  SaturateOnIntegerOverflow=on
  Data Type Conversion1 : DataTypeConversion  DataType=double  SaturateOnIntegerOverflow=on
  Relational Operator : RelationalOperator  Operator=>  InputSameDT=on
  Out : Outport
  wires:
  Relational Operator/1 -> Out/1  "bit 0"
  Bitwise Logical Operator/1 -> Data Type Conversion1/1
  Constant1/1 -> Relational Operator/2
  Data Type Conversion/1 -> Bitwise Logical Operator/1
  In/1 -> Data Type Conversion/1
  Data Type Conversion1/1 -> Relational Operator/1

== system WiFi_lib/11Mbps demod/Integer to binary/bit 1 ==
  In : Inport
  Bitwise Logical Operator : simulink3/Math/Bitwise Logical Operator  Operator=AND  Operand2=2
  Constant1 : Constant  Value=0
  Data Type Conversion : DataTypeConversion  DataType=uint8  SaturateOnIntegerOverflow=on
  Data Type Conversion1 : DataTypeConversion  DataType=double  SaturateOnIntegerOverflow=on
  Relational Operator : RelationalOperator  Operator=>  InputSameDT=on
  Out : Outport
  wires:
  Data Type Conversion1/1 -> Relational Operator/1
  In/1 -> Data Type Conversion/1
  Data Type Conversion/1 -> Bitwise Logical Operator/1
  Constant1/1 -> Relational Operator/2
  Bitwise Logical Operator/1 -> Data Type Conversion1/1
  Relational Operator/1 -> Out/1  "bit 0"

== system WiFi_lib/11Mbps demod/Integer to binary/bit 2 ==
  In : Inport
  Bitwise Logical Operator : simulink3/Math/Bitwise Logical Operator  Operator=AND  Operand2=4
  Constant1 : Constant  Value=0
  Data Type Conversion : DataTypeConversion  DataType=uint8  SaturateOnIntegerOverflow=on
  Data Type Conversion1 : DataTypeConversion  DataType=double  SaturateOnIntegerOverflow=on
  Relational Operator : RelationalOperator  Operator=>  InputSameDT=on
  Out : Outport
  wires:
  Relational Operator/1 -> Out/1  "bit 0"
  Bitwise Logical Operator/1 -> Data Type Conversion1/1
  Constant1/1 -> Relational Operator/2
  Data Type Conversion/1 -> Bitwise Logical Operator/1
  In/1 -> Data Type Conversion/1
  Data Type Conversion1/1 -> Relational Operator/1

== system WiFi_lib/11Mbps demod/Integer to binary/bit 3 ==
  In : Inport
  Bitwise Logical Operator : simulink3/Math/Bitwise Logical Operator  Operator=AND  Operand2=8
  Constant1 : Constant  Value=0
  Data Type Conversion : DataTypeConversion  DataType=uint8  SaturateOnIntegerOverflow=on
  Data Type Conversion1 : DataTypeConversion  DataType=double  SaturateOnIntegerOverflow=on
  Relational Operator : RelationalOperator  Operator=>  InputSameDT=on
  Out : Outport
  wires:
  Data Type Conversion1/1 -> Relational Operator/1
  In/1 -> Data Type Conversion/1
  Data Type Conversion/1 -> Bitwise Logical Operator/1
  Constant1/1 -> Relational Operator/2
  Bitwise Logical Operator/1 -> Data Type Conversion1/1
  Relational Operator/1 -> Out/1  "bit 0"

== system WiFi_lib/11Mbps demod/Integer to binary/bit 4 ==
  In : Inport
  Bitwise Logical Operator : simulink3/Math/Bitwise Logical Operator  Operator=AND  Operand2=16
  Constant1 : Constant  Value=0
  Data Type Conversion : DataTypeConversion  DataType=uint8  SaturateOnIntegerOverflow=on
  Data Type Conversion1 : DataTypeConversion  DataType=double  SaturateOnIntegerOverflow=on
  Relational Operator : RelationalOperator  Operator=>  InputSameDT=on
  Out : Outport
  wires:
  Relational Operator/1 -> Out/1  "bit 0"
  Bitwise Logical Operator/1 -> Data Type Conversion1/1
  Constant1/1 -> Relational Operator/2
  Data Type Conversion/1 -> Bitwise Logical Operator/1
  In/1 -> Data Type Conversion/1
  Data Type Conversion1/1 -> Relational Operator/1

== system WiFi_lib/11Mbps demod/Integer to binary/bit 5 ==
  In : Inport
  Bitwise Logical Operator : simulink3/Math/Bitwise Logical Operator  Operator=AND  Operand2=32
  Constant1 : Constant  Value=0
  Data Type Conversion : DataTypeConversion  DataType=uint8  SaturateOnIntegerOverflow=on
  Data Type Conversion1 : DataTypeConversion  DataType=double  SaturateOnIntegerOverflow=on
  Relational Operator : RelationalOperator  Operator=>  InputSameDT=on
  Out : Outport
  wires:
  Data Type Conversion1/1 -> Relational Operator/1
  In/1 -> Data Type Conversion/1
  Data Type Conversion/1 -> Bitwise Logical Operator/1
  Constant1/1 -> Relational Operator/2
  Bitwise Logical Operator/1 -> Data Type Conversion1/1
  Relational Operator/1 -> Out/1  "bit 0"

== system WiFi_lib/5.5Mbps demod/Integer to binary/bit 0 ==
  In : Inport
  Bitwise Logical Operator : simulink3/Math/Bitwise Logical Operator  Operator=AND  Operand2=1
  Constant1 : Constant  Value=0
  Data Type Conversion : DataTypeConversion  DataType=uint8  SaturateOnIntegerOverflow=on
  Data Type Conversion1 : DataTypeConversion  DataType=double  SaturateOnIntegerOverflow=on
  Relational Operator : RelationalOperator  Operator=>  InputSameDT=on
  Out : Outport
  wires:
  Data Type Conversion1/1 -> Relational Operator/1
  In/1 -> Data Type Conversion/1
  Data Type Conversion/1 -> Bitwise Logical Operator/1
  Constant1/1 -> Relational Operator/2
  Bitwise Logical Operator/1 -> Data Type Conversion1/1
  Relational Operator/1 -> Out/1  "bit 0"

== system WiFi_lib/5.5Mbps demod/Integer to binary/bit 1 ==
  In : Inport
  Bitwise Logical Operator : simulink3/Math/Bitwise Logical Operator  Operator=AND  Operand2=2
  Constant1 : Constant  Value=0
  Data Type Conversion : DataTypeConversion  DataType=uint8  SaturateOnIntegerOverflow=on
  Data Type Conversion1 : DataTypeConversion  DataType=double  SaturateOnIntegerOverflow=on
  Relational Operator : RelationalOperator  Operator=>  InputSameDT=on
  Out : Outport
  wires:
  Relational Operator/1 -> Out/1  "bit 0"
  Bitwise Logical Operator/1 -> Data Type Conversion1/1
  Constant1/1 -> Relational Operator/2
  Data Type Conversion/1 -> Bitwise Logical Operator/1
  In/1 -> Data Type Conversion/1
  Data Type Conversion1/1 -> Relational Operator/1
